simulink model "soru2"  (R2025b)
settings: Solver=VariableStepAuto  StartTime=0.0  StopTime=10.0  RelTol=1e-3
settings Model: Creator=Seyma  LastModifiedBy=Seyma

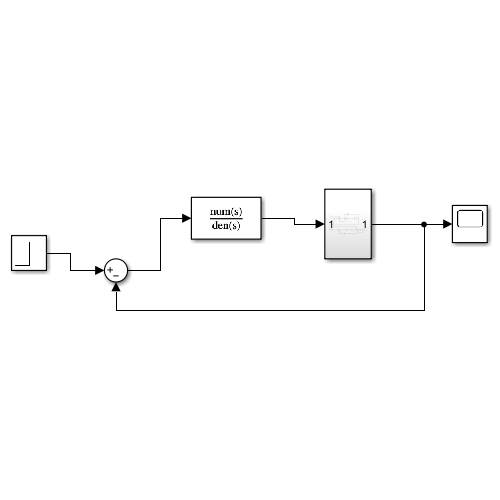
[thumbnail: Simulink's stored preview of the top-level diagram]
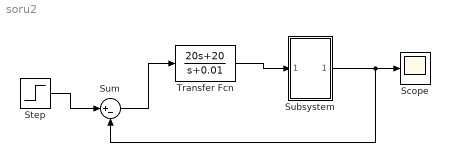
== system soru2 ==
  Scope : Scope
      settings: ActiveDisplayYMinimum=-0.18450275022195969  ActiveDisplayYMaximum=1.6605247519976376
  Step : Step  Time=0  SampleTime=0
  Subsystem : Subsystem
  Sum : Sum  Inputs=|+-
  Transfer Fcn : TransferFcn  Numerator=[20 20]  Denominator=[1 0.01]
  wires:
  Subsystem/1(Out1) -> Sum/2, Scope/1
  Step/1 -> Sum/1
  Sum/1 -> Transfer Fcn/1
  Transfer Fcn/1 -> Subsystem/1(In1)

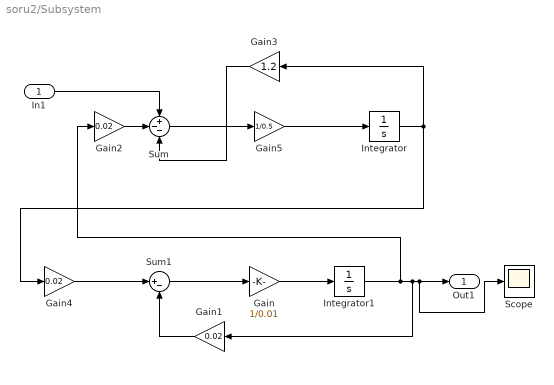
== system soru2/Subsystem ==
  In1 : Inport
  Gain : Gain  Gain=1/0.01
  Gain1 : Gain  Gain=0.02
  Gain2 : Gain  Gain=0.02
  Gain3 : Gain  Gain=1.2
  Gain4 : Gain  Gain=0.02
  Gain5 : Gain  Gain=1/0.5
  Integrator : Integrator
  Integrator1 : Integrator
  Scope : Scope
      settings: ActiveDisplayYMinimum=-1  ActiveDisplayYMaximum=1
  Sum : Sum  Inputs=+--
  Sum1 : Sum  Inputs=|+-
  Out1 : Outport
  wires:
  Gain2/1 -> Sum/2
  Sum1/1 -> Gain/1
  Gain5/1 -> Integrator/1
  Integrator/1 -> Gain3/1, Gain4/1
  Gain3/1 -> Sum/3
  Gain1/1 -> Sum1/2
  Sum/1 -> Gain5/1
  Integrator1/1 -> Gain2/1, Gain1/1, Out1/1, Scope/1
  Gain/1 -> Integrator1/1
  Gain4/1 -> Sum1/1
  In1/1 -> Sum/1
